simulink model "PoissonKinematics"  (R2023a)
settings: Solver=VariableStepAuto  StartTime=0.0  StopTime=100.0  RelTol=1e-3
undefined symbols (not defined in the file): Cnb0, pitch, roll, yaw
settings Model: Creator=prafulsigdel  LastModifiedBy=prafulsigdel

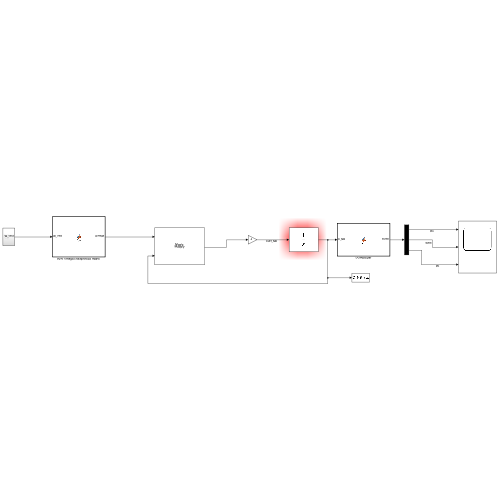
[thumbnail: Simulink's stored preview of the top-level diagram]
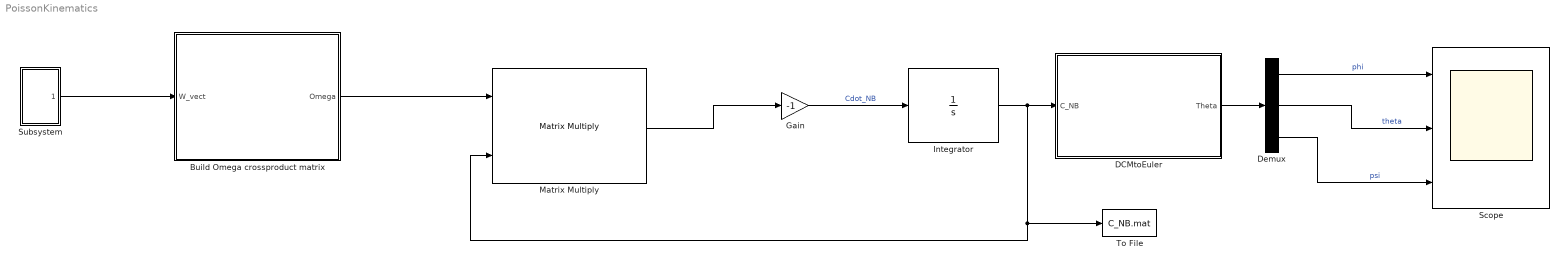
== system PoissonKinematics ==
  "Build Omega crossproduct matrix " : MATLAB Function  TreatAsAtomicUnit=on
  DCMtoEuler : MATLAB Function  TreatAsAtomicUnit=on
  Demux : Demux  Outputs=3
  Gain : Gain  Gain=-1
  Integrator : Integrator  InitialCondition=Cnb0
  Matrix Multiply : Product  Multiplication=Matrix(*)
  Scope : Scope  NumInputPorts=3
  Subsystem : Subsystem
  To File : ToFile  Filename=C_NB.mat  SaveFormat=Timeseries
  wires:
  Subsystem/1(W_vect) -> "Build Omega crossproduct matrix "/1(W_vect)
  "Build Omega crossproduct matrix "/1(Omega) -> Matrix Multiply/1
  Matrix Multiply/1 -> Gain/1
  Gain/1 -> Integrator/1  "Cdot_NB"
  Integrator/1 -> To File/1, Matrix Multiply/2, DCMtoEuler/1(C_NB)
  DCMtoEuler/1(Theta) -> Demux/1
  Demux/1 -> Scope/1  "phi"
  Demux/2 -> Scope/2  "theta"
  Demux/3 -> Scope/3  "psi"

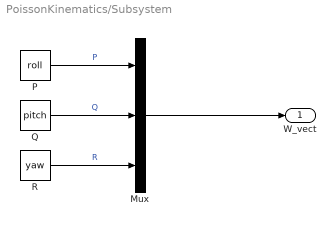
== system PoissonKinematics/Subsystem ==
  Mux : Mux  Inputs=3
  P : Constant  Value=roll
  Q : Constant  Value=pitch
  R : Constant  Value=yaw
  W_vect : Outport
  wires:
  P/1 -> Mux/1  "P"
  R/1 -> Mux/3  "R"
  Q/1 -> Mux/2  "Q"
  Mux/1 -> W_vect/1

== matlab function PoissonKinematics/Build Omega crossproduct matrix  ==
  data: W_vect input; Omega output
function Omega = fcn(W_vect)

p = W_vect(1);
q = W_vect(2);
r = W_vect(3);


Omega = [0 -r q;
    r 0 -p;
    -q p 0];

== matlab function PoissonKinematics/DCMtoEuler ==
  data: C_NB input; Theta output
function Theta = fcn(C_NB)

c11 = C_NB(1,1);
c12 = C_NB(1,2);
c13 = C_NB(1,3);
c23 = C_NB(2,3);
c33 = C_NB(3,3);

roll = atan2(c23,c33);
pitch = -asin(c13);
yaw = atan2(c12,c11);

Theta = [roll;pitch;yaw];
